simulink model "LQR"  (R2019b)
settings: Solver=VariableStepAuto  StartTime=0.0  StopTime=50  RelTol=1e-3
values from neighbouring files (symbols this model uses):
  Ad = sysd.A    [lqr.m]
  Bd = sysd.B    [lqr.m]
undefined symbols (not defined in the file or in its folder): Klqr
settings Model: Creator=Martin  LastModifiedBy=krthk

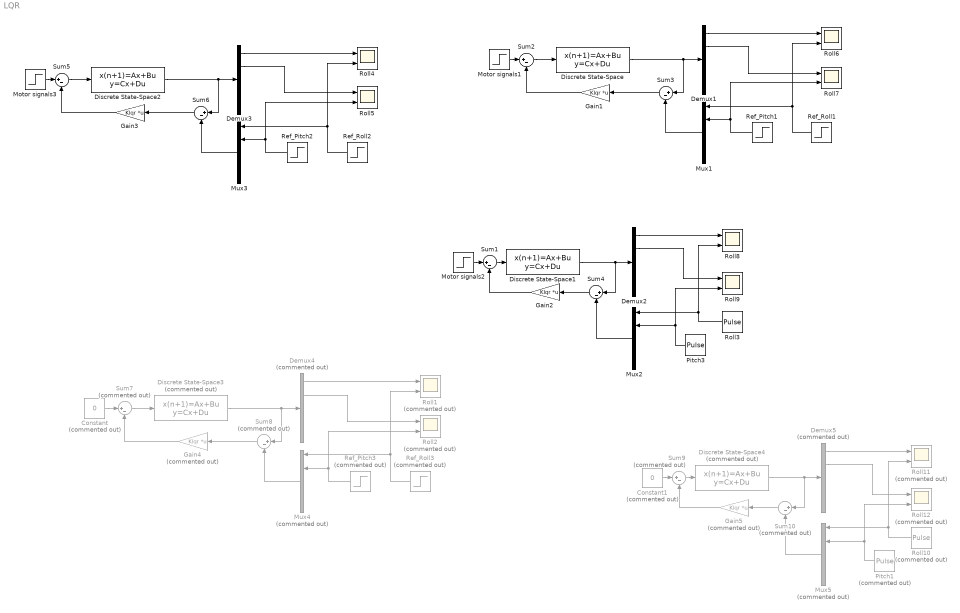
== system LQR ==
  Constant : Constant  Commented=on  Value=0
  Constant1 : Constant  Commented=on  Value=0
  Demux1 : Demux  Outputs=5
  Demux2 : Demux  Outputs=5
  Demux3 : Demux  Outputs=5
  Demux4 : Demux  Commented=on  Outputs=5
  Demux5 : Demux  Commented=on  Outputs=5
  Discrete State-Space : DiscreteStateSpace  A=Ad  B=Bd  C=eye(5)  D=zeros(5,4)  SampleTime=0.01
  Discrete State-Space1 : DiscreteStateSpace  A=Ad  B=Bd  C=eye(5)  D=zeros(5,4)  SampleTime=0.01
  Discrete State-Space2 : DiscreteStateSpace  A=Ad  B=Bd  C=eye(5)  D=zeros(5,4)  SampleTime=0.01
  Discrete State-Space3 : DiscreteStateSpace  Commented=on  A=Ad  B=Bd  C=eye(5)  D=zeros(5,4)  SampleTime=0.01
  Discrete State-Space4 : DiscreteStateSpace  Commented=on  A=Ad  B=Bd  C=eye(5)  D=zeros(5,4)  SampleTime=0.01
  Gain1 : Gain  Gain=Klqr  Multiplication=Matrix(K*u)
  Gain2 : Gain  Gain=Klqr  Multiplication=Matrix(K*u)
  Gain3 : Gain  Gain=Klqr  Multiplication=Matrix(K*u)
  Gain4 : Gain  Commented=on  Gain=Klqr  Multiplication=Matrix(K*u)
  Gain5 : Gain  Commented=on  Gain=Klqr  Multiplication=Matrix(K*u)
  Motor signals1 : Step  After=[0; 0; 0; 0]  SampleTime=20
  Motor signals2 : Step  After=[0; 0; 0; 0]  SampleTime=20
  Motor signals3 : Step  After=[0; 0; 0; 0]  SampleTime=20
  Mux1 : Mux  Inputs=5
  Mux2 : Mux  Inputs=5
  Mux3 : Mux  Inputs=5
  Mux4 : Mux  Commented=on  Inputs=5
  Mux5 : Mux  Commented=on  Inputs=5
  Pitch1 : DiscretePulseGenerator  Commented=on  PulseType=Time based  Amplitude=6  Period=100  PulseWidth=0.5  PhaseDelay=5
  Pitch3 : DiscretePulseGenerator  PulseType=Time based  Amplitude=6  Period=100  PulseWidth=0.5  PhaseDelay=5
  Ref_Pitch1 : Step  Time=20  Before=10  After=0  SampleTime=0
  Ref_Pitch2 : Step  Time=20  After=10  SampleTime=0
  Ref_Pitch3 : Step  Commented=on  Time=20  After=10  SampleTime=0
  Ref_Roll1 : Step  Time=20  Before=10  After=0  SampleTime=0
  Ref_Roll2 : Step  Time=20  After=10  SampleTime=0
  Ref_Roll3 : Step  Commented=on  Time=20  After=10  SampleTime=0
  Roll{1..2,11..12} (4 alike) : Scope  Commented=on  NumInputPorts=2
  Roll10 : DiscretePulseGenerator  Commented=on  PulseType=Time based  Amplitude=6  Period=100  PulseWidth=0.5  PhaseDelay=5
  Roll3 : DiscretePulseGenerator  PulseType=Time based  Amplitude=6  Period=100  PulseWidth=0.5  PhaseDelay=5
  Roll{4..9} (6 alike) : Scope  NumInputPorts=2
  Sum{1..6} (6 alike) : Sum  Inputs=|+-
  Sum{7..10} (4 alike) : Sum  Commented=on  Inputs=|+-
  wires:
  Sum2/1 -> Discrete State-Space/1
  Sum3/1 -> Gain1/1
  Mux1/1 -> Sum3/2
  Gain1/1 -> Sum2/2
  Motor signals1/1 -> Sum2/1
  Demux1/2 -> Roll7/1
  Discrete State-Space/1 -> Demux1/1, Sum3/1
  Demux1/1 -> Roll6/1
  Discrete State-Space1/1 -> Sum4/1, Demux2/1
  Demux2/1 -> Roll8/1
  Roll3/1 -> Roll8/2, Mux2/1
  Gain2/1 -> Sum1/2
  Mux2/1 -> Sum4/2
  Sum4/1 -> Gain2/1
  Demux2/2 -> Roll9/1
  Sum1/1 -> Discrete State-Space1/1
  Motor signals2/1 -> Sum1/1
  Ref_Roll1/1 -> Roll6/2, Mux1/1
  Ref_Pitch1/1 -> Roll7/2, Mux1/2
  Pitch3/1 -> Roll9/2, Mux2/2
  Ref_Pitch2/1 -> Roll5/2, Mux3/2
  Ref_Roll2/1 -> Mux3/1, Roll4/2
  Demux3/1 -> Roll4/1
  Gain3/1 -> Sum5/2
  Mux3/1 -> Sum6/2
  Sum6/1 -> Gain3/1
  Demux3/2 -> Roll5/1
  Discrete State-Space2/1 -> Demux3/1, Sum6/1
  Sum5/1 -> Discrete State-Space2/1
  Motor signals3/1 -> Sum5/1
  Demux4/2 -> Roll2/1
  Sum7/1 -> Discrete State-Space3/1
  Discrete State-Space3/1 -> Demux4/1, Sum8/1
  Gain4/1 -> Sum7/2
  Sum8/1 -> Gain4/1
  Constant/1 -> Sum7/1
  Mux4/1 -> Sum8/2
  Ref_Roll3/1 -> Mux4/1, Roll1/2
  Ref_Pitch3/1 -> Roll2/2, Mux4/2
  Demux4/1 -> Roll1/1
  Pitch1/1 -> Roll12/2, Mux5/2
  Demux5/1 -> Roll11/1
  Discrete State-Space4/1 -> Sum10/1, Demux5/1
  Demux5/2 -> Roll12/1
  Sum10/1 -> Gain5/1
  Mux5/1 -> Sum10/2
  Constant1/1 -> Sum9/1
  Gain5/1 -> Sum9/2
  Roll10/1 -> Roll11/2, Mux5/1
  Sum9/1 -> Discrete State-Space4/1
